simulink model "P_Furuta_LQRG"  (R2016b)
settings: Solver=ode45  StartTime=0.0  StopTime=10  RelTol=1e-3
values from neighbouring files (symbols this model uses):
  M1 = MK(:,1)    [Linealizacion_LQRG.m]    (also in Linealizacion_LQRG_Integrador.m = MKi(:,1))
  M2 = MK(:,2)    [Linealizacion_LQRG.m]    (also in Linealizacion_LQRG_Integrador.m = MKi(:,2))
  M3 = MK(:,3)    [Linealizacion_LQRG.m]    (also in Linealizacion_LQRG_Integrador.m = MKi(:,3))
  M4 = MK(:,4)    [Linealizacion_LQRG.m]    (also in Linealizacion_LQRG_Integrador.m = MKi(:,4))
  Rango = -20*(0.0175):0.0175:20*(0.0175)    [Linealizacion_LQRG.m]    (also in Linealizacion_LQRG_Integrador.m)
undefined symbols (not defined in the file or in its folder): magnitude
settings Model: Creator=eq  LastModifiedBy=eq
settings DataIOCC: LimitDataPoints=on  SaveFormat=Array
settings OptimizationCC: BlockReduction=off  BooleanDataType=off  LifeSpan=inf
settings DebuggingCC: SaveWithParameterizedLinksMsg=none  UnderspecifiedInitializationDetection=Classic  MergeDetectMultiDrivingBlocksExec=none  SignalResolutionControl=TryResolveAllWithWarning  SFUnexpectedBacktrackingDiag=warning  SFNoUnconditionalDefaultTransitionDiag=warning  SFExecutionAtInitializationDiag=none
settings HardwareCC: ProdBitPerPointer=32  ProdBitPerSizeT=32  ProdBitPerPtrDiffT=32  ProdLargestAtomicFloat=None  ProdIntDivRoundTo=Undefined  ProdEndianess=Unspecified  ProdWordSize=32  ProdHWDeviceType=32-bit Generic  TargetUnknown=on
settings ModelReferenceCC: PropagateSignalLabelsOutOfModel=off
settings GRTTargetCC: TargetLangStandard=C89/C90 (ANSI)  GeneratePreprocessorConditionals=Disable all
settings ConfigComp: CovMetricSettings=dw  CovHtmlReporting=on  CovSaveCumulativeToWorkspaceVar=on  CovSaveSingleToWorkspaceVar=on  CovExternalEMLEnable=off  CovSFcnEnable=off

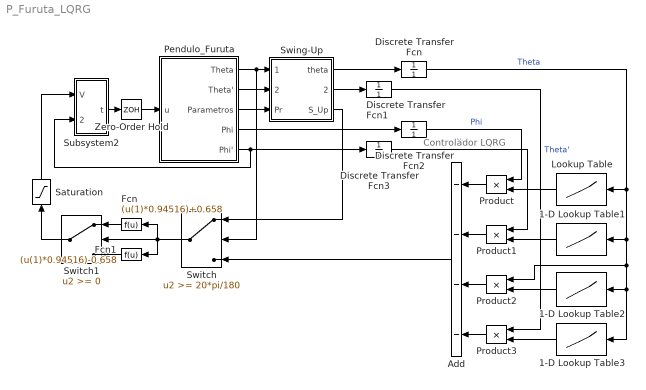
== system P_Furuta_LQRG ==
  note: Controlador LQRG
  1-D Lookup Table1 : Lookup_n-D  NumberOfTableDimensions=1  BreakpointsForDimension1=Rango  Table=M2  InternalRulePriority=Speed  RndMeth=Simplest  InputSameDT=on
  1-D Lookup Table2 : Lookup_n-D  NumberOfTableDimensions=1  BreakpointsForDimension1=Rango  Table=M3  InternalRulePriority=Speed  RndMeth=Simplest  InputSameDT=on
  1-D Lookup Table3 : Lookup_n-D  NumberOfTableDimensions=1  BreakpointsForDimension1=Rango  Table=M4  InternalRulePriority=Speed  RndMeth=Simplest  InputSameDT=on
  Add : Sum  Inputs=----
  Discrete Transfer Fcn{,1..3} (4 alike) : DiscreteTransferFcn  Denominator=[1]  SampleTime=0.01
  Fcn : Fcn  Expr=(u(1)*0.94516)+0.658
  Fcn1 : Fcn  Expr=(u(1)*0.94516)-0.658
  Lookup Table : Lookup_n-D  NumberOfTableDimensions=1  BreakpointsForDimension1=Rango  Table=M1  InternalRulePriority=Speed  RndMeth=Simplest  InputSameDT=on
  Pendulo_Furuta : Subsystem  mask{mp=0.015, lp=0.2, mb=0.245, lb=0.15, J=0.0023146, g=9.8}
      mask prompts: mp "Masa_Pendulo(Kg)"; lp "Longitud_Pendulo(m)"; mb "Masa_Brazo(Kg)"; lb "Longitud_Brazo(m)"; J "Inercia"; g "Gravedad(m/s^2)"
  Product{,1..3} (4 alike) : Product
  Saturation : Saturate  UpperLimit=5  LowerLimit=-5
  Subsystem2 : Subsystem  mask{Ke=0.353, R=2.34, Kt=0.15}
  Swing-Up : Subsystem
  Switch : Switch  Threshold=20*pi/180
  Switch1 : Switch
  Zero-Order Hold : ZeroOrderHold  SampleTime=0.01
  wires:
  Swing-Up/3(S_Up) -> Switch/1
  Pendulo_Furuta/1(Theta) -> Swing-Up/1(Theta), Switch/2
  Pendulo_Furuta/2(Theta') -> Swing-Up/2(Theta')
  Swing-Up/2(theta') -> Discrete Transfer Fcn1/1
  Pendulo_Furuta/5(Phi') -> Discrete Transfer Fcn3/1, Subsystem2/2("Phi' ")
  Swing-Up/1(theta) -> Discrete Transfer Fcn/1
  Pendulo_Furuta/4(Phi) -> Discrete Transfer Fcn2/1
  Subsystem2/1("t ") -> Zero-Order Hold/1
  Zero-Order Hold/1 -> Pendulo_Furuta/1(u)
  Discrete Transfer Fcn2/1 -> Product/1  "Phi"
  Discrete Transfer Fcn/1 -> Product2/1, 1-D Lookup Table2/1, 1-D Lookup Table3/1, 1-D Lookup Table1/1, Lookup Table/1  "Theta"
  Add/1 -> Switch/3
  Lookup Table/1 -> Product/2
  Product/1 -> Add/1
  Product1/1 -> Add/2
  1-D Lookup Table1/1 -> Product1/2
  Product2/1 -> Add/3
  1-D Lookup Table2/1 -> Product2/2
  Product3/1 -> Add/4
  1-D Lookup Table3/1 -> Product3/2
  Discrete Transfer Fcn1/1 -> Product3/1  "Theta'"
  Switch/1 -> Fcn1/1, Fcn/1, Switch1/2
  Fcn/1 -> Switch1/1
  Fcn1/1 -> Switch1/3
  Switch1/1 -> Saturation/1
  Saturation/1 -> Subsystem2/1(V)
  Pendulo_Furuta/3(Parametros) -> Swing-Up/3(Pr)
  Discrete Transfer Fcn3/1 -> Product1/1  "Phi'"

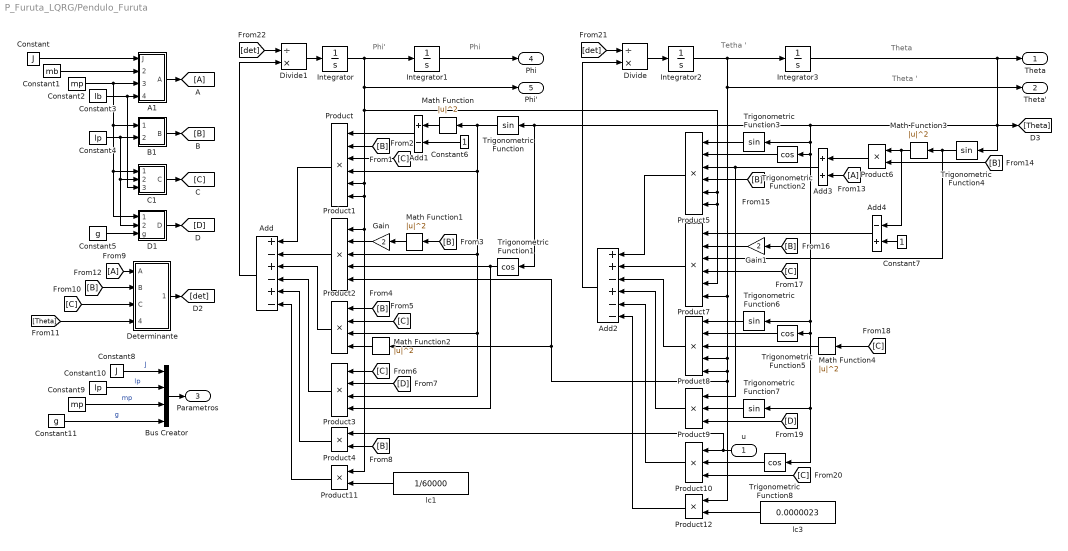
== system P_Furuta_LQRG/Pendulo_Furuta ==
  note: Phi
  note: Phi'
  note: Theta
  note: Tetha '
  note: Theta '
  u : Inport
  A1 : Subsystem
  Add : Sum  Inputs=+-+-+-
  Add1 : Sum  Inputs=+-
  Add2 : Sum  Inputs=++-+--
  Add3 : Sum
  Add4 : Sum  Inputs=-+
  B1 : Subsystem
  Bus Creator : BusCreator  Inputs=4
  C1 : Subsystem
  Constant : Constant  Value=J
  Constant1 : Constant  Value=mb
  Constant10 : Constant  Value=lp
  Constant11 : Constant  Value=g
  Constant2 : Constant  Value=mp
  Constant3 : Constant  Value=lb
  Constant4 : Constant  Value=lp
  Constant5 : Constant  Value=g
  Constant6 : Constant
  Constant7 : Constant
  Constant8 : Constant  Value=J
  Constant9 : Constant  Value=mp
  D1 : Subsystem
  Determinante : Subsystem
  Divide : Product  Inputs=/*
  Divide1 : Product  Inputs=/*
  Gain : Gain  Gain=2
  Gain1 : Gain  Gain=2
  Integrator : Integrator
  Integrator1 : Integrator
  Integrator2 : Integrator
  Integrator3 : Integrator  InitialCondition=pi
  Math Function{,1..4} (5 alike) : Math  Operator=magnitude^2  SaturateOnIntegerOverflow=on
  Product : Product  Inputs=6
  Product1 : Product  Inputs=5
  Product10 : Product  Inputs=3
  Product{4,6,11..12} (4 alike) : Product
  Product2 : Product  Inputs=4
  Product3 : Product  Inputs=4
  Product5 : Product  Inputs=6
  Product7 : Product  Inputs=6
  Product8 : Product  Inputs=5
  Product9 : Product  Inputs=3
  Trigonometric Function{,3..4,6..7} (5 alike) : Trigonometry
  Trigonometric Function{1..2,5,8} (4 alike) : Trigonometry  Operator=cos
  lc1 : Constant  Value=1/60000
  lc3 : Constant  Value=0.0000023
  Theta : Outport
  Theta' : Outport  Port=2
  Parametros : Outport  Port=3
  Phi : Outport  Port=4
  Phi' : Outport  Port=5
  wires:
  B1/1("B ") -> [B]
  [D] -> Product3/2
  Constant4/1 -> B1/2(lp), C1/2(lp), D1/2(lp)
  D1/1("D ") -> [D]
  Constant2/1 -> A1/3(mp), B1/1(mp), D1/1(mp), C1/1(mp)
  Constant5/1 -> D1/3(g)
  Determinante/1(det) -> [det]
  Math Function2/1 -> Product2/4
  Integrator/1 -> Integrator1/1, Phi'/1, Product7/5, Product5/6, Product5/5, Product/5, Product11/1, Product1/1, Product/6
  Gain/1 -> Product1/2
  Trigonometric Function1/1 -> Product3/4, Product1/4
  A1/1(A) -> [A]
  [B] -> Math Function1/1
  C1/1("C ") -> [C]
  [A] -> Determinante/1(A)
  Constant1/1 -> A1/2(mb)
  Integrator2/1 -> Integrator3/1, Theta'/1, Product12/1, Product1/5, Math Function2/1, Product8/5, Product8/4, Product7/6
  [C] -> Product3/1
  [C] -> Product2/2
  Integrator1/1 -> Phi/1
  Constant3/1 -> C1/3(lb), A1/4(lb)
  Integrator3/1 -> Theta/1, Trigonometric Function4/1, [Theta], Trigonometric Function1/1, Trigonometric Function/1, Trigonometric Function6/1, Trigonometric Function8/1, Trigonometric Function7/1, Trigonometric Function5/1, Trigonometric Function2/1, Trigonometric Function3/1
  Math Function1/1 -> Gain/1
  Trigonometric Function/1 -> Math Function/1, Product/4, Product1/3, Product2/3, Product3/3
  [C] -> Determinante/3(C)
  [B] -> Product2/1
  [Theta] -> Determinante/4("Tetha ")
  [B] -> Determinante/2(B)
  [B] -> Product/2
  [C] -> Product/3
  Add1/1 -> Product/1
  Constant6/1 -> Add1/2
  Math Function/1 -> Add1/1
  Trigonometric Function3/1 -> Product5/1
  Trigonometric Function2/1 -> Product5/2
  Add3/1 -> Product9/1, Product5/3
  [A] -> Add3/2
  Product6/1 -> Add3/1
  Math Function3/1 -> Add4/1, Product6/1
  Trigonometric Function4/1 -> Product7/3, Math Function3/1
  [B] -> Product6/2
  [B] -> Product5/4
  Constant7/1 -> Add4/2
  Add4/1 -> Product7/1
  [B] -> Gain1/1
  Gain1/1 -> Product7/2
  [C] -> Product7/4
  Trigonometric Function5/1 -> Product8/2
  Math Function4/1 -> Product8/3
  [C] -> Math Function4/1
  Trigonometric Function6/1 -> Product8/1
  Trigonometric Function7/1 -> Product9/2
  [D] -> Product9/3
  Trigonometric Function8/1 -> Product10/2
  [C] -> Product10/3
  u/1 -> Product4/1, Product10/1
  [B] -> Product4/2
  Divide/1 -> Integrator2/1
  Divide1/1 -> Integrator/1
  Product/1 -> Add/1
  Product1/1 -> Add/2
  Product2/1 -> Add/3
  Product3/1 -> Add/4
  Product4/1 -> Add/5
  [det] -> Divide1/1
  Add/1 -> Divide1/2
  [det] -> Divide/1
  Add2/1 -> Divide/2
  Product5/1 -> Add2/1
  Product7/1 -> Add2/2
  Product8/1 -> Add2/3
  Product9/1 -> Add2/4
  Product10/1 -> Add2/5
  Bus Creator/1 -> Parametros/1
  Constant/1 -> A1/1(J)
  Constant11/1 -> Bus Creator/4  "g"
  Constant8/1 -> Bus Creator/1  "J"
  lc1/1 -> Product11/2
  lc3/1 -> Product12/2
  Product11/1 -> Add/6
  Product12/1 -> Add2/6
  Constant10/1 -> Bus Creator/2  "lp"
  Constant9/1 -> Bus Creator/3  "mp"

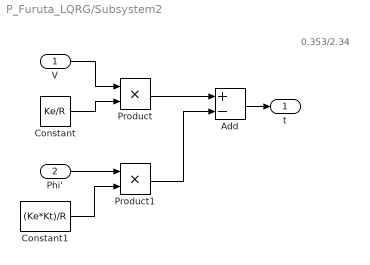
== system P_Furuta_LQRG/Subsystem2 ==
  note: 0.353/2.34
  V : Inport
  "Phi' " : Inport  Port=2
  Add : Sum  Inputs=+-
  Constant : Constant  Value=Ke/R
  Constant1 : Constant  Value=(Ke*Kt)/R
  Product : Product
  Product1 : Product
  "t " : Outport
  wires:
  V/1 -> Product/1
  Constant/1 -> Product/2
  Product/1 -> Add/1
  Product1/1 -> Add/2
  "Phi' "/1 -> Product1/1
  Constant1/1 -> Product1/2
  Add/1 -> "t "/1

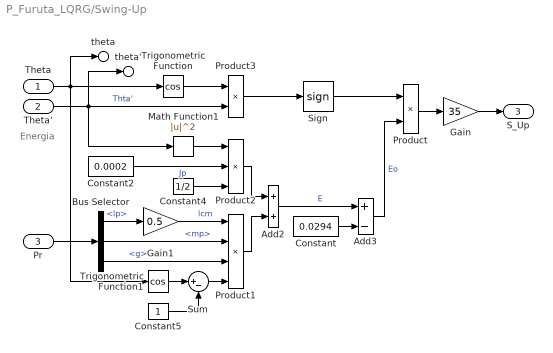
== system P_Furuta_LQRG/Swing-Up ==
  note: Energia
  Theta : Inport
  Theta' : Inport  Port=2
  Pr : Inport  Port=3
  Add2 : Sum
  Add3 : Sum  Inputs=+-
  Bus Selector : BusSelector  OutputSignals=lp,mp,g
  Constant : Constant  Value=0.0294
  Constant2 : Constant  Value=0.0002
  Constant4 : Constant  Value=1/2
  Constant5 : Constant
  Gain : Gain  Gain=35
  Gain1 : Gain  Gain=0.5
  Math Function1 : Math  Operator=magnitude^2  SaturateOnIntegerOverflow=on
  Product : Product
  Product1 : Product  Inputs=4
  Product2 : Product  Inputs=3
  Product3 : Product
  Sign : Signum
  Sum : Sum  Inputs=|+-
  Trigonometric Function : Trigonometry  Operator=cos
  Trigonometric Function1 : Trigonometry  Operator=cos
  theta : Outport
  theta' : Outport  Port=2
  S_Up : Outport  Port=3
  wires:
  Trigonometric Function/1 -> Product3/1
  Theta'/1 -> theta'/1, Product3/2, Math Function1/1  "Thta'"
  Product3/1 -> Sign/1
  Pr/1 -> Bus Selector/1
  Bus Selector/2 -> Product1/2  "<mp>"
  Bus Selector/1 -> Gain1/1  "<lp>"
  Constant2/1 -> Product2/2  "Jp"
  Constant4/1 -> Product2/3
  Bus Selector/3 -> Product1/3  "<g>"
  Trigonometric Function1/1 -> Sum/1
  Constant5/1 -> Sum/2
  Product1/1 -> Add2/2
  Add2/1 -> Add3/1  "E"
  Sign/1 -> Product/1
  Product/1 -> Gain/1
  Constant/1 -> Add3/2
  Gain/1 -> S_Up/1
  Product2/1 -> Add2/1
  Theta/1 -> theta/1, Trigonometric Function1/1, Trigonometric Function/1
  Add3/1 -> Product/2  "Eo"
  Sum/1 -> Product1/4
  Gain1/1 -> Product1/1  "lcm"
  Math Function1/1 -> Product2/1

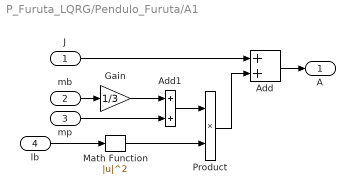
== system P_Furuta_LQRG/Pendulo_Furuta/A1 ==
  J : Inport
  mb : Inport  Port=2
  mp : Inport  Port=3
  lb : Inport  Port=4
  Add : Sum
  Add1 : Sum
  Gain : Gain  Gain=1/3
  Math Function : Math  Operator=magnitude^2  SaturateOnIntegerOverflow=on
  Product : Product
  A : Outport
  wires:
  Add1/1 -> Product/1
  Product/1 -> Add/2
  Add/1 -> A/1
  J/1 -> Add/1
  mb/1 -> Gain/1
  mp/1 -> Add1/2
  Gain/1 -> Add1/1
  lb/1 -> Math Function/1
  Math Function/1 -> Product/2

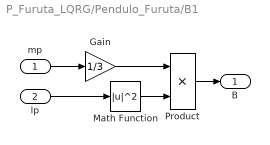
== system P_Furuta_LQRG/Pendulo_Furuta/B1 ==
  mp : Inport
  lp : Inport  Port=2
  Gain : Gain  Gain=1/3
  Math Function : Math  Operator=magnitude^2  SaturateOnIntegerOverflow=on
  Product : Product
  "B " : Outport
  wires:
  Product/1 -> "B "/1
  mp/1 -> Gain/1
  lp/1 -> Math Function/1
  Gain/1 -> Product/1
  Math Function/1 -> Product/2

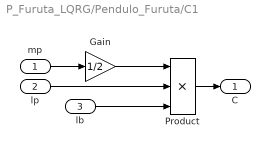
== system P_Furuta_LQRG/Pendulo_Furuta/C1 ==
  mp : Inport
  lp : Inport  Port=2
  lb : Inport  Port=3
  Gain : Gain  Gain=1/2
  Product : Product  Inputs=3
  "C " : Outport
  wires:
  Product/1 -> "C "/1
  mp/1 -> Gain/1
  Gain/1 -> Product/1
  lp/1 -> Product/2
  lb/1 -> Product/3

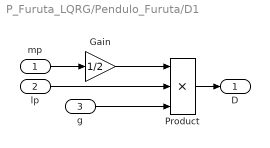
== system P_Furuta_LQRG/Pendulo_Furuta/D1 ==
  mp : Inport
  lp : Inport  Port=2
  g : Inport  Port=3
  Gain : Gain  Gain=1/2
  Product : Product  Inputs=3
  "D " : Outport
  wires:
  Product/1 -> "D "/1
  mp/1 -> Gain/1
  Gain/1 -> Product/1
  lp/1 -> Product/2
  g/1 -> Product/3

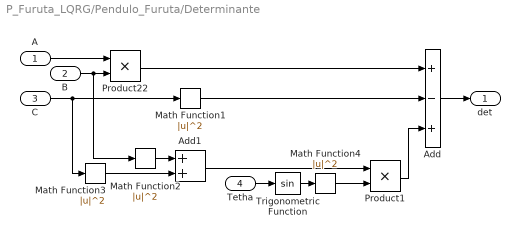
== system P_Furuta_LQRG/Pendulo_Furuta/Determinante ==
  A : Inport
  B : Inport  Port=2
  C : Inport  Port=3
  "Tetha " : Inport  Port=4
  Add : Sum  Inputs=+-+
  Add1 : Sum
  Math Function{1..4} (4 alike) : Math  Operator=magnitude^2  SaturateOnIntegerOverflow=on
  Product1 : Product
  Product22 : Product
  Trigonometric Function : Trigonometry
  det : Outport
  wires:
  A/1 -> Product22/1
  B/1 -> Math Function2/1, Product22/2
  Product22/1 -> Add/1
  C/1 -> Math Function3/1, Math Function1/1
  Math Function1/1 -> Add/2
  "Tetha "/1 -> Trigonometric Function/1
  Add1/1 -> Product1/1
  Math Function2/1 -> Add1/1
  Math Function3/1 -> Add1/2
  Trigonometric Function/1 -> Math Function4/1
  Math Function4/1 -> Product1/2
  Product1/1 -> Add/3
  Add/1 -> det/1
